simulink model "gm_parallel_lht"  (R2019b)
settings: Solver=FixedStepDiscrete  StartTime=0.0  StopTime=inf  RelTol=1e-3
undefined symbols (not defined in the file or in its folder): bt, height, width
libraries: hdlsllib x190, simulink x13, hdlmdlgenlib x7, dspsrcs4 x1
(part 15 of 18)

== system gm_parallel_lht/Parallel LHT/Parallel LHT Accumulator/Accumulator with Switches/Accumulator_instance35/Block RAM/Simple Dual Port RAM ==
  wr_data : Inport  OutDataTypeStr=fixdt(0, 11, 0)  PortDimensions=1  SampleTime=6.66666666666667e-09
  wr_addr : Inport  Port=2  OutDataTypeStr=fixdt(0, 11, 0)  PortDimensions=1  SampleTime=6.66666666666667e-09
  wr_en : Inport  Port=3  OutDataTypeStr=boolean  PortDimensions=1  SampleTime=6.66666666666667e-09
  rd_addr : Inport  Port=4  OutDataTypeStr=fixdt(0, 11, 0)  PortDimensions=1  SampleTime=6.66666666666667e-09
  Simple Dual Port RAM : hdlsllib/HDL RAMs/Simple Dual Port RAM  ram_size=ceil(log2(maxRho*2))
      settings: SourceProductName=Simulink  SourceProductBaseCode=SL
  rd_data : Outport
  wires:
  rd_addr/1 -> Simple Dual Port RAM/4
  wr_en/1 -> Simple Dual Port RAM/3
  wr_addr/1 -> Simple Dual Port RAM/2
  wr_data/1 -> Simple Dual Port RAM/1
  Simple Dual Port RAM/1 -> rd_data/1

== system gm_parallel_lht/Parallel LHT/Parallel LHT Accumulator/Accumulator with Switches/Accumulator_instance36/Block RAM/Simple Dual Port RAM ==
  wr_data : Inport  OutDataTypeStr=fixdt(0, 11, 0)  PortDimensions=1  SampleTime=6.66666666666667e-09
  wr_addr : Inport  Port=2  OutDataTypeStr=fixdt(0, 11, 0)  PortDimensions=1  SampleTime=6.66666666666667e-09
  wr_en : Inport  Port=3  OutDataTypeStr=boolean  PortDimensions=1  SampleTime=6.66666666666667e-09
  rd_addr : Inport  Port=4  OutDataTypeStr=fixdt(0, 11, 0)  PortDimensions=1  SampleTime=6.66666666666667e-09
  Simple Dual Port RAM : hdlsllib/HDL RAMs/Simple Dual Port RAM  ram_size=ceil(log2(maxRho*2))
      settings: SourceProductName=Simulink  SourceProductBaseCode=SL
  rd_data : Outport
  wires:
  rd_addr/1 -> Simple Dual Port RAM/4
  wr_en/1 -> Simple Dual Port RAM/3
  wr_addr/1 -> Simple Dual Port RAM/2
  wr_data/1 -> Simple Dual Port RAM/1
  Simple Dual Port RAM/1 -> rd_data/1

== system gm_parallel_lht/Parallel LHT/Parallel LHT Accumulator/Accumulator with Switches/Accumulator_instance37/Block RAM/Simple Dual Port RAM ==
  wr_data : Inport  OutDataTypeStr=fixdt(0, 11, 0)  PortDimensions=1  SampleTime=6.66666666666667e-09
  wr_addr : Inport  Port=2  OutDataTypeStr=fixdt(0, 11, 0)  PortDimensions=1  SampleTime=6.66666666666667e-09
  wr_en : Inport  Port=3  OutDataTypeStr=boolean  PortDimensions=1  SampleTime=6.66666666666667e-09
  rd_addr : Inport  Port=4  OutDataTypeStr=fixdt(0, 11, 0)  PortDimensions=1  SampleTime=6.66666666666667e-09
  Simple Dual Port RAM : hdlsllib/HDL RAMs/Simple Dual Port RAM  ram_size=ceil(log2(maxRho*2))
      settings: SourceProductName=Simulink  SourceProductBaseCode=SL
  rd_data : Outport
  wires:
  rd_addr/1 -> Simple Dual Port RAM/4
  wr_en/1 -> Simple Dual Port RAM/3
  wr_addr/1 -> Simple Dual Port RAM/2
  wr_data/1 -> Simple Dual Port RAM/1
  Simple Dual Port RAM/1 -> rd_data/1

== system gm_parallel_lht/Parallel LHT/Parallel LHT Accumulator/Accumulator with Switches/Accumulator_instance38/Block RAM/Simple Dual Port RAM ==
  wr_data : Inport  OutDataTypeStr=fixdt(0, 11, 0)  PortDimensions=1  SampleTime=6.66666666666667e-09
  wr_addr : Inport  Port=2  OutDataTypeStr=fixdt(0, 11, 0)  PortDimensions=1  SampleTime=6.66666666666667e-09
  wr_en : Inport  Port=3  OutDataTypeStr=boolean  PortDimensions=1  SampleTime=6.66666666666667e-09
  rd_addr : Inport  Port=4  OutDataTypeStr=fixdt(0, 11, 0)  PortDimensions=1  SampleTime=6.66666666666667e-09
  Simple Dual Port RAM : hdlsllib/HDL RAMs/Simple Dual Port RAM  ram_size=ceil(log2(maxRho*2))
      settings: SourceProductName=Simulink  SourceProductBaseCode=SL
  rd_data : Outport
  wires:
  rd_addr/1 -> Simple Dual Port RAM/4
  wr_en/1 -> Simple Dual Port RAM/3
  wr_addr/1 -> Simple Dual Port RAM/2
  wr_data/1 -> Simple Dual Port RAM/1
  Simple Dual Port RAM/1 -> rd_data/1

== system gm_parallel_lht/Parallel LHT/Parallel LHT Accumulator/Accumulator with Switches/Accumulator_instance39/Block RAM/Simple Dual Port RAM ==
  wr_data : Inport  OutDataTypeStr=fixdt(0, 11, 0)  PortDimensions=1  SampleTime=6.66666666666667e-09
  wr_addr : Inport  Port=2  OutDataTypeStr=fixdt(0, 11, 0)  PortDimensions=1  SampleTime=6.66666666666667e-09
  wr_en : Inport  Port=3  OutDataTypeStr=boolean  PortDimensions=1  SampleTime=6.66666666666667e-09
  rd_addr : Inport  Port=4  OutDataTypeStr=fixdt(0, 11, 0)  PortDimensions=1  SampleTime=6.66666666666667e-09
  Simple Dual Port RAM : hdlsllib/HDL RAMs/Simple Dual Port RAM  ram_size=ceil(log2(maxRho*2))
      settings: SourceProductName=Simulink  SourceProductBaseCode=SL
  rd_data : Outport
  wires:
  rd_addr/1 -> Simple Dual Port RAM/4
  wr_en/1 -> Simple Dual Port RAM/3
  wr_addr/1 -> Simple Dual Port RAM/2
  wr_data/1 -> Simple Dual Port RAM/1
  Simple Dual Port RAM/1 -> rd_data/1

== system gm_parallel_lht/Parallel LHT/Parallel LHT Accumulator/Accumulator with Switches/Accumulator_instance4/Block RAM/Simple Dual Port RAM ==
  wr_data : Inport  OutDataTypeStr=fixdt(0, 11, 0)  PortDimensions=1  SampleTime=6.66666666666667e-09
  wr_addr : Inport  Port=2  OutDataTypeStr=fixdt(0, 11, 0)  PortDimensions=1  SampleTime=6.66666666666667e-09
  wr_en : Inport  Port=3  OutDataTypeStr=boolean  PortDimensions=1  SampleTime=6.66666666666667e-09
  rd_addr : Inport  Port=4  OutDataTypeStr=fixdt(0, 11, 0)  PortDimensions=1  SampleTime=6.66666666666667e-09
  Simple Dual Port RAM : hdlsllib/HDL RAMs/Simple Dual Port RAM  ram_size=ceil(log2(maxRho*2))
      settings: SourceProductName=Simulink  SourceProductBaseCode=SL
  rd_data : Outport
  wires:
  rd_addr/1 -> Simple Dual Port RAM/4
  wr_en/1 -> Simple Dual Port RAM/3
  wr_addr/1 -> Simple Dual Port RAM/2
  wr_data/1 -> Simple Dual Port RAM/1
  Simple Dual Port RAM/1 -> rd_data/1

== system gm_parallel_lht/Parallel LHT/Parallel LHT Accumulator/Accumulator with Switches/Accumulator_instance40/Block RAM/Simple Dual Port RAM ==
  wr_data : Inport  OutDataTypeStr=fixdt(0, 11, 0)  PortDimensions=1  SampleTime=6.66666666666667e-09
  wr_addr : Inport  Port=2  OutDataTypeStr=fixdt(0, 11, 0)  PortDimensions=1  SampleTime=6.66666666666667e-09
  wr_en : Inport  Port=3  OutDataTypeStr=boolean  PortDimensions=1  SampleTime=6.66666666666667e-09
  rd_addr : Inport  Port=4  OutDataTypeStr=fixdt(0, 11, 0)  PortDimensions=1  SampleTime=6.66666666666667e-09
  Simple Dual Port RAM : hdlsllib/HDL RAMs/Simple Dual Port RAM  ram_size=ceil(log2(maxRho*2))
      settings: SourceProductName=Simulink  SourceProductBaseCode=SL
  rd_data : Outport
  wires:
  rd_addr/1 -> Simple Dual Port RAM/4
  wr_en/1 -> Simple Dual Port RAM/3
  wr_addr/1 -> Simple Dual Port RAM/2
  wr_data/1 -> Simple Dual Port RAM/1
  Simple Dual Port RAM/1 -> rd_data/1

== system gm_parallel_lht/Parallel LHT/Parallel LHT Accumulator/Accumulator with Switches/Accumulator_instance41/Block RAM/Simple Dual Port RAM ==
  wr_data : Inport  OutDataTypeStr=fixdt(0, 11, 0)  PortDimensions=1  SampleTime=6.66666666666667e-09
  wr_addr : Inport  Port=2  OutDataTypeStr=fixdt(0, 11, 0)  PortDimensions=1  SampleTime=6.66666666666667e-09
  wr_en : Inport  Port=3  OutDataTypeStr=boolean  PortDimensions=1  SampleTime=6.66666666666667e-09
  rd_addr : Inport  Port=4  OutDataTypeStr=fixdt(0, 11, 0)  PortDimensions=1  SampleTime=6.66666666666667e-09
  Simple Dual Port RAM : hdlsllib/HDL RAMs/Simple Dual Port RAM  ram_size=ceil(log2(maxRho*2))
      settings: SourceProductName=Simulink  SourceProductBaseCode=SL
  rd_data : Outport
  wires:
  rd_addr/1 -> Simple Dual Port RAM/4
  wr_en/1 -> Simple Dual Port RAM/3
  wr_addr/1 -> Simple Dual Port RAM/2
  wr_data/1 -> Simple Dual Port RAM/1
  Simple Dual Port RAM/1 -> rd_data/1

== system gm_parallel_lht/Parallel LHT/Parallel LHT Accumulator/Accumulator with Switches/Accumulator_instance42/Block RAM/Simple Dual Port RAM ==
  wr_data : Inport  OutDataTypeStr=fixdt(0, 11, 0)  PortDimensions=1  SampleTime=6.66666666666667e-09
  wr_addr : Inport  Port=2  OutDataTypeStr=fixdt(0, 11, 0)  PortDimensions=1  SampleTime=6.66666666666667e-09
  wr_en : Inport  Port=3  OutDataTypeStr=boolean  PortDimensions=1  SampleTime=6.66666666666667e-09
  rd_addr : Inport  Port=4  OutDataTypeStr=fixdt(0, 11, 0)  PortDimensions=1  SampleTime=6.66666666666667e-09
  Simple Dual Port RAM : hdlsllib/HDL RAMs/Simple Dual Port RAM  ram_size=ceil(log2(maxRho*2))
      settings: SourceProductName=Simulink  SourceProductBaseCode=SL
  rd_data : Outport
  wires:
  rd_addr/1 -> Simple Dual Port RAM/4
  wr_en/1 -> Simple Dual Port RAM/3
  wr_addr/1 -> Simple Dual Port RAM/2
  wr_data/1 -> Simple Dual Port RAM/1
  Simple Dual Port RAM/1 -> rd_data/1

== system gm_parallel_lht/Parallel LHT/Parallel LHT Accumulator/Accumulator with Switches/Accumulator_instance43/Block RAM/Simple Dual Port RAM ==
  wr_data : Inport  OutDataTypeStr=fixdt(0, 11, 0)  PortDimensions=1  SampleTime=6.66666666666667e-09
  wr_addr : Inport  Port=2  OutDataTypeStr=fixdt(0, 11, 0)  PortDimensions=1  SampleTime=6.66666666666667e-09
  wr_en : Inport  Port=3  OutDataTypeStr=boolean  PortDimensions=1  SampleTime=6.66666666666667e-09
  rd_addr : Inport  Port=4  OutDataTypeStr=fixdt(0, 11, 0)  PortDimensions=1  SampleTime=6.66666666666667e-09
  Simple Dual Port RAM : hdlsllib/HDL RAMs/Simple Dual Port RAM  ram_size=ceil(log2(maxRho*2))
      settings: SourceProductName=Simulink  SourceProductBaseCode=SL
  rd_data : Outport
  wires:
  rd_addr/1 -> Simple Dual Port RAM/4
  wr_en/1 -> Simple Dual Port RAM/3
  wr_addr/1 -> Simple Dual Port RAM/2
  wr_data/1 -> Simple Dual Port RAM/1
  Simple Dual Port RAM/1 -> rd_data/1

== system gm_parallel_lht/Parallel LHT/Parallel LHT Accumulator/Accumulator with Switches/Accumulator_instance44/Block RAM/Simple Dual Port RAM ==
  wr_data : Inport  OutDataTypeStr=fixdt(0, 11, 0)  PortDimensions=1  SampleTime=6.66666666666667e-09
  wr_addr : Inport  Port=2  OutDataTypeStr=fixdt(0, 11, 0)  PortDimensions=1  SampleTime=6.66666666666667e-09
  wr_en : Inport  Port=3  OutDataTypeStr=boolean  PortDimensions=1  SampleTime=6.66666666666667e-09
  rd_addr : Inport  Port=4  OutDataTypeStr=fixdt(0, 11, 0)  PortDimensions=1  SampleTime=6.66666666666667e-09
  Simple Dual Port RAM : hdlsllib/HDL RAMs/Simple Dual Port RAM  ram_size=ceil(log2(maxRho*2))
      settings: SourceProductName=Simulink  SourceProductBaseCode=SL
  rd_data : Outport
  wires:
  rd_addr/1 -> Simple Dual Port RAM/4
  wr_en/1 -> Simple Dual Port RAM/3
  wr_addr/1 -> Simple Dual Port RAM/2
  wr_data/1 -> Simple Dual Port RAM/1
  Simple Dual Port RAM/1 -> rd_data/1

== system gm_parallel_lht/Parallel LHT/Parallel LHT Accumulator/Accumulator with Switches/Accumulator_instance45/Block RAM/Simple Dual Port RAM ==
  wr_data : Inport  OutDataTypeStr=fixdt(0, 11, 0)  PortDimensions=1  SampleTime=6.66666666666667e-09
  wr_addr : Inport  Port=2  OutDataTypeStr=fixdt(0, 11, 0)  PortDimensions=1  SampleTime=6.66666666666667e-09
  wr_en : Inport  Port=3  OutDataTypeStr=boolean  PortDimensions=1  SampleTime=6.66666666666667e-09
  rd_addr : Inport  Port=4  OutDataTypeStr=fixdt(0, 11, 0)  PortDimensions=1  SampleTime=6.66666666666667e-09
  Simple Dual Port RAM : hdlsllib/HDL RAMs/Simple Dual Port RAM  ram_size=ceil(log2(maxRho*2))
      settings: SourceProductName=Simulink  SourceProductBaseCode=SL
  rd_data : Outport
  wires:
  rd_addr/1 -> Simple Dual Port RAM/4
  wr_en/1 -> Simple Dual Port RAM/3
  wr_addr/1 -> Simple Dual Port RAM/2
  wr_data/1 -> Simple Dual Port RAM/1
  Simple Dual Port RAM/1 -> rd_data/1

== system gm_parallel_lht/Parallel LHT/Parallel LHT Accumulator/Accumulator with Switches/Accumulator_instance46/Block RAM/Simple Dual Port RAM ==
  wr_data : Inport  OutDataTypeStr=fixdt(0, 11, 0)  PortDimensions=1  SampleTime=6.66666666666667e-09
  wr_addr : Inport  Port=2  OutDataTypeStr=fixdt(0, 11, 0)  PortDimensions=1  SampleTime=6.66666666666667e-09
  wr_en : Inport  Port=3  OutDataTypeStr=boolean  PortDimensions=1  SampleTime=6.66666666666667e-09
  rd_addr : Inport  Port=4  OutDataTypeStr=fixdt(0, 11, 0)  PortDimensions=1  SampleTime=6.66666666666667e-09
  Simple Dual Port RAM : hdlsllib/HDL RAMs/Simple Dual Port RAM  ram_size=ceil(log2(maxRho*2))
      settings: SourceProductName=Simulink  SourceProductBaseCode=SL
  rd_data : Outport
  wires:
  rd_addr/1 -> Simple Dual Port RAM/4
  wr_en/1 -> Simple Dual Port RAM/3
  wr_addr/1 -> Simple Dual Port RAM/2
  wr_data/1 -> Simple Dual Port RAM/1
  Simple Dual Port RAM/1 -> rd_data/1

== system gm_parallel_lht/Parallel LHT/Parallel LHT Accumulator/Accumulator with Switches/Accumulator_instance47/Block RAM/Simple Dual Port RAM ==
  wr_data : Inport  OutDataTypeStr=fixdt(0, 11, 0)  PortDimensions=1  SampleTime=6.66666666666667e-09
  wr_addr : Inport  Port=2  OutDataTypeStr=fixdt(0, 11, 0)  PortDimensions=1  SampleTime=6.66666666666667e-09
  wr_en : Inport  Port=3  OutDataTypeStr=boolean  PortDimensions=1  SampleTime=6.66666666666667e-09
  rd_addr : Inport  Port=4  OutDataTypeStr=fixdt(0, 11, 0)  PortDimensions=1  SampleTime=6.66666666666667e-09
  Simple Dual Port RAM : hdlsllib/HDL RAMs/Simple Dual Port RAM  ram_size=ceil(log2(maxRho*2))
      settings: SourceProductName=Simulink  SourceProductBaseCode=SL
  rd_data : Outport
  wires:
  rd_addr/1 -> Simple Dual Port RAM/4
  wr_en/1 -> Simple Dual Port RAM/3
  wr_addr/1 -> Simple Dual Port RAM/2
  wr_data/1 -> Simple Dual Port RAM/1
  Simple Dual Port RAM/1 -> rd_data/1

== system gm_parallel_lht/Parallel LHT/Parallel LHT Accumulator/Accumulator with Switches/Accumulator_instance48/Block RAM/Simple Dual Port RAM ==
  wr_data : Inport  OutDataTypeStr=fixdt(0, 11, 0)  PortDimensions=1  SampleTime=6.66666666666667e-09
  wr_addr : Inport  Port=2  OutDataTypeStr=fixdt(0, 11, 0)  PortDimensions=1  SampleTime=6.66666666666667e-09
  wr_en : Inport  Port=3  OutDataTypeStr=boolean  PortDimensions=1  SampleTime=6.66666666666667e-09
  rd_addr : Inport  Port=4  OutDataTypeStr=fixdt(0, 11, 0)  PortDimensions=1  SampleTime=6.66666666666667e-09
  Simple Dual Port RAM : hdlsllib/HDL RAMs/Simple Dual Port RAM  ram_size=ceil(log2(maxRho*2))
      settings: SourceProductName=Simulink  SourceProductBaseCode=SL
  rd_data : Outport
  wires:
  rd_addr/1 -> Simple Dual Port RAM/4
  wr_en/1 -> Simple Dual Port RAM/3
  wr_addr/1 -> Simple Dual Port RAM/2
  wr_data/1 -> Simple Dual Port RAM/1
  Simple Dual Port RAM/1 -> rd_data/1

== system gm_parallel_lht/Parallel LHT/Parallel LHT Accumulator/Accumulator with Switches/Accumulator_instance49/Block RAM/Simple Dual Port RAM ==
  wr_data : Inport  OutDataTypeStr=fixdt(0, 11, 0)  PortDimensions=1  SampleTime=6.66666666666667e-09
  wr_addr : Inport  Port=2  OutDataTypeStr=fixdt(0, 11, 0)  PortDimensions=1  SampleTime=6.66666666666667e-09
  wr_en : Inport  Port=3  OutDataTypeStr=boolean  PortDimensions=1  SampleTime=6.66666666666667e-09
  rd_addr : Inport  Port=4  OutDataTypeStr=fixdt(0, 11, 0)  PortDimensions=1  SampleTime=6.66666666666667e-09
  Simple Dual Port RAM : hdlsllib/HDL RAMs/Simple Dual Port RAM  ram_size=ceil(log2(maxRho*2))
      settings: SourceProductName=Simulink  SourceProductBaseCode=SL
  rd_data : Outport
  wires:
  rd_addr/1 -> Simple Dual Port RAM/4
  wr_en/1 -> Simple Dual Port RAM/3
  wr_addr/1 -> Simple Dual Port RAM/2
  wr_data/1 -> Simple Dual Port RAM/1
  Simple Dual Port RAM/1 -> rd_data/1

== system gm_parallel_lht/Parallel LHT/Parallel LHT Accumulator/Accumulator with Switches/Accumulator_instance5/Block RAM/Simple Dual Port RAM ==
  wr_data : Inport  OutDataTypeStr=fixdt(0, 11, 0)  PortDimensions=1  SampleTime=6.66666666666667e-09
  wr_addr : Inport  Port=2  OutDataTypeStr=fixdt(0, 11, 0)  PortDimensions=1  SampleTime=6.66666666666667e-09
  wr_en : Inport  Port=3  OutDataTypeStr=boolean  PortDimensions=1  SampleTime=6.66666666666667e-09
  rd_addr : Inport  Port=4  OutDataTypeStr=fixdt(0, 11, 0)  PortDimensions=1  SampleTime=6.66666666666667e-09
  Simple Dual Port RAM : hdlsllib/HDL RAMs/Simple Dual Port RAM  ram_size=ceil(log2(maxRho*2))
      settings: SourceProductName=Simulink  SourceProductBaseCode=SL
  rd_data : Outport
  wires:
  rd_addr/1 -> Simple Dual Port RAM/4
  wr_en/1 -> Simple Dual Port RAM/3
  wr_addr/1 -> Simple Dual Port RAM/2
  wr_data/1 -> Simple Dual Port RAM/1
  Simple Dual Port RAM/1 -> rd_data/1

== system gm_parallel_lht/Parallel LHT/Parallel LHT Accumulator/Accumulator with Switches/Accumulator_instance50/Block RAM/Simple Dual Port RAM ==
  wr_data : Inport  OutDataTypeStr=fixdt(0, 11, 0)  PortDimensions=1  SampleTime=6.66666666666667e-09
  wr_addr : Inport  Port=2  OutDataTypeStr=fixdt(0, 11, 0)  PortDimensions=1  SampleTime=6.66666666666667e-09
  wr_en : Inport  Port=3  OutDataTypeStr=boolean  PortDimensions=1  SampleTime=6.66666666666667e-09
  rd_addr : Inport  Port=4  OutDataTypeStr=fixdt(0, 11, 0)  PortDimensions=1  SampleTime=6.66666666666667e-09
  Simple Dual Port RAM : hdlsllib/HDL RAMs/Simple Dual Port RAM  ram_size=ceil(log2(maxRho*2))
      settings: SourceProductName=Simulink  SourceProductBaseCode=SL
  rd_data : Outport
  wires:
  rd_addr/1 -> Simple Dual Port RAM/4
  wr_en/1 -> Simple Dual Port RAM/3
  wr_addr/1 -> Simple Dual Port RAM/2
  wr_data/1 -> Simple Dual Port RAM/1
  Simple Dual Port RAM/1 -> rd_data/1

== system gm_parallel_lht/Parallel LHT/Parallel LHT Accumulator/Accumulator with Switches/Accumulator_instance51/Block RAM/Simple Dual Port RAM ==
  wr_data : Inport  OutDataTypeStr=fixdt(0, 11, 0)  PortDimensions=1  SampleTime=6.66666666666667e-09
  wr_addr : Inport  Port=2  OutDataTypeStr=fixdt(0, 11, 0)  PortDimensions=1  SampleTime=6.66666666666667e-09
  wr_en : Inport  Port=3  OutDataTypeStr=boolean  PortDimensions=1  SampleTime=6.66666666666667e-09
  rd_addr : Inport  Port=4  OutDataTypeStr=fixdt(0, 11, 0)  PortDimensions=1  SampleTime=6.66666666666667e-09
  Simple Dual Port RAM : hdlsllib/HDL RAMs/Simple Dual Port RAM  ram_size=ceil(log2(maxRho*2))
      settings: SourceProductName=Simulink  SourceProductBaseCode=SL
  rd_data : Outport
  wires:
  rd_addr/1 -> Simple Dual Port RAM/4
  wr_en/1 -> Simple Dual Port RAM/3
  wr_addr/1 -> Simple Dual Port RAM/2
  wr_data/1 -> Simple Dual Port RAM/1
  Simple Dual Port RAM/1 -> rd_data/1

== system gm_parallel_lht/Parallel LHT/Parallel LHT Accumulator/Accumulator with Switches/Accumulator_instance52/Block RAM/Simple Dual Port RAM ==
  wr_data : Inport  OutDataTypeStr=fixdt(0, 11, 0)  PortDimensions=1  SampleTime=6.66666666666667e-09
  wr_addr : Inport  Port=2  OutDataTypeStr=fixdt(0, 11, 0)  PortDimensions=1  SampleTime=6.66666666666667e-09
  wr_en : Inport  Port=3  OutDataTypeStr=boolean  PortDimensions=1  SampleTime=6.66666666666667e-09
  rd_addr : Inport  Port=4  OutDataTypeStr=fixdt(0, 11, 0)  PortDimensions=1  SampleTime=6.66666666666667e-09
  Simple Dual Port RAM : hdlsllib/HDL RAMs/Simple Dual Port RAM  ram_size=ceil(log2(maxRho*2))
      settings: SourceProductName=Simulink  SourceProductBaseCode=SL
  rd_data : Outport
  wires:
  rd_addr/1 -> Simple Dual Port RAM/4
  wr_en/1 -> Simple Dual Port RAM/3
  wr_addr/1 -> Simple Dual Port RAM/2
  wr_data/1 -> Simple Dual Port RAM/1
  Simple Dual Port RAM/1 -> rd_data/1

== system gm_parallel_lht/Parallel LHT/Parallel LHT Accumulator/Accumulator with Switches/Accumulator_instance53/Block RAM/Simple Dual Port RAM ==
  wr_data : Inport  OutDataTypeStr=fixdt(0, 11, 0)  PortDimensions=1  SampleTime=6.66666666666667e-09
  wr_addr : Inport  Port=2  OutDataTypeStr=fixdt(0, 11, 0)  PortDimensions=1  SampleTime=6.66666666666667e-09
  wr_en : Inport  Port=3  OutDataTypeStr=boolean  PortDimensions=1  SampleTime=6.66666666666667e-09
  rd_addr : Inport  Port=4  OutDataTypeStr=fixdt(0, 11, 0)  PortDimensions=1  SampleTime=6.66666666666667e-09
  Simple Dual Port RAM : hdlsllib/HDL RAMs/Simple Dual Port RAM  ram_size=ceil(log2(maxRho*2))
      settings: SourceProductName=Simulink  SourceProductBaseCode=SL
  rd_data : Outport
  wires:
  rd_addr/1 -> Simple Dual Port RAM/4
  wr_en/1 -> Simple Dual Port RAM/3
  wr_addr/1 -> Simple Dual Port RAM/2
  wr_data/1 -> Simple Dual Port RAM/1
  Simple Dual Port RAM/1 -> rd_data/1

== system gm_parallel_lht/Parallel LHT/Parallel LHT Accumulator/Accumulator with Switches/Accumulator_instance54/Block RAM/Simple Dual Port RAM ==
  wr_data : Inport  OutDataTypeStr=fixdt(0, 11, 0)  PortDimensions=1  SampleTime=6.66666666666667e-09
  wr_addr : Inport  Port=2  OutDataTypeStr=fixdt(0, 11, 0)  PortDimensions=1  SampleTime=6.66666666666667e-09
  wr_en : Inport  Port=3  OutDataTypeStr=boolean  PortDimensions=1  SampleTime=6.66666666666667e-09
  rd_addr : Inport  Port=4  OutDataTypeStr=fixdt(0, 11, 0)  PortDimensions=1  SampleTime=6.66666666666667e-09
  Simple Dual Port RAM : hdlsllib/HDL RAMs/Simple Dual Port RAM  ram_size=ceil(log2(maxRho*2))
      settings: SourceProductName=Simulink  SourceProductBaseCode=SL
  rd_data : Outport
  wires:
  rd_addr/1 -> Simple Dual Port RAM/4
  wr_en/1 -> Simple Dual Port RAM/3
  wr_addr/1 -> Simple Dual Port RAM/2
  wr_data/1 -> Simple Dual Port RAM/1
  Simple Dual Port RAM/1 -> rd_data/1

== system gm_parallel_lht/Parallel LHT/Parallel LHT Accumulator/Accumulator with Switches/Accumulator_instance55/Block RAM/Simple Dual Port RAM ==
  wr_data : Inport  OutDataTypeStr=fixdt(0, 11, 0)  PortDimensions=1  SampleTime=6.66666666666667e-09
  wr_addr : Inport  Port=2  OutDataTypeStr=fixdt(0, 11, 0)  PortDimensions=1  SampleTime=6.66666666666667e-09
  wr_en : Inport  Port=3  OutDataTypeStr=boolean  PortDimensions=1  SampleTime=6.66666666666667e-09
  rd_addr : Inport  Port=4  OutDataTypeStr=fixdt(0, 11, 0)  PortDimensions=1  SampleTime=6.66666666666667e-09
  Simple Dual Port RAM : hdlsllib/HDL RAMs/Simple Dual Port RAM  ram_size=ceil(log2(maxRho*2))
      settings: SourceProductName=Simulink  SourceProductBaseCode=SL
  rd_data : Outport
  wires:
  rd_addr/1 -> Simple Dual Port RAM/4
  wr_en/1 -> Simple Dual Port RAM/3
  wr_addr/1 -> Simple Dual Port RAM/2
  wr_data/1 -> Simple Dual Port RAM/1
  Simple Dual Port RAM/1 -> rd_data/1

== system gm_parallel_lht/Parallel LHT/Parallel LHT Accumulator/Accumulator with Switches/Accumulator_instance56/Block RAM/Simple Dual Port RAM ==
  wr_data : Inport  OutDataTypeStr=fixdt(0, 11, 0)  PortDimensions=1  SampleTime=6.66666666666667e-09
  wr_addr : Inport  Port=2  OutDataTypeStr=fixdt(0, 11, 0)  PortDimensions=1  SampleTime=6.66666666666667e-09
  wr_en : Inport  Port=3  OutDataTypeStr=boolean  PortDimensions=1  SampleTime=6.66666666666667e-09
  rd_addr : Inport  Port=4  OutDataTypeStr=fixdt(0, 11, 0)  PortDimensions=1  SampleTime=6.66666666666667e-09
  Simple Dual Port RAM : hdlsllib/HDL RAMs/Simple Dual Port RAM  ram_size=ceil(log2(maxRho*2))
      settings: SourceProductName=Simulink  SourceProductBaseCode=SL
  rd_data : Outport
  wires:
  rd_addr/1 -> Simple Dual Port RAM/4
  wr_en/1 -> Simple Dual Port RAM/3
  wr_addr/1 -> Simple Dual Port RAM/2
  wr_data/1 -> Simple Dual Port RAM/1
  Simple Dual Port RAM/1 -> rd_data/1

== system gm_parallel_lht/Parallel LHT/Parallel LHT Accumulator/Accumulator with Switches/Accumulator_instance57/Block RAM/Simple Dual Port RAM ==
  wr_data : Inport  OutDataTypeStr=fixdt(0, 11, 0)  PortDimensions=1  SampleTime=6.66666666666667e-09
  wr_addr : Inport  Port=2  OutDataTypeStr=fixdt(0, 11, 0)  PortDimensions=1  SampleTime=6.66666666666667e-09
  wr_en : Inport  Port=3  OutDataTypeStr=boolean  PortDimensions=1  SampleTime=6.66666666666667e-09
  rd_addr : Inport  Port=4  OutDataTypeStr=fixdt(0, 11, 0)  PortDimensions=1  SampleTime=6.66666666666667e-09
  Simple Dual Port RAM : hdlsllib/HDL RAMs/Simple Dual Port RAM  ram_size=ceil(log2(maxRho*2))
      settings: SourceProductName=Simulink  SourceProductBaseCode=SL
  rd_data : Outport
  wires:
  rd_addr/1 -> Simple Dual Port RAM/4
  wr_en/1 -> Simple Dual Port RAM/3
  wr_addr/1 -> Simple Dual Port RAM/2
  wr_data/1 -> Simple Dual Port RAM/1
  Simple Dual Port RAM/1 -> rd_data/1

== system gm_parallel_lht/Parallel LHT/Parallel LHT Accumulator/Accumulator with Switches/Accumulator_instance58/Block RAM/Simple Dual Port RAM ==
  wr_data : Inport  OutDataTypeStr=fixdt(0, 11, 0)  PortDimensions=1  SampleTime=6.66666666666667e-09
  wr_addr : Inport  Port=2  OutDataTypeStr=fixdt(0, 11, 0)  PortDimensions=1  SampleTime=6.66666666666667e-09
  wr_en : Inport  Port=3  OutDataTypeStr=boolean  PortDimensions=1  SampleTime=6.66666666666667e-09
  rd_addr : Inport  Port=4  OutDataTypeStr=fixdt(0, 11, 0)  PortDimensions=1  SampleTime=6.66666666666667e-09
  Simple Dual Port RAM : hdlsllib/HDL RAMs/Simple Dual Port RAM  ram_size=ceil(log2(maxRho*2))
      settings: SourceProductName=Simulink  SourceProductBaseCode=SL
  rd_data : Outport
  wires:
  rd_addr/1 -> Simple Dual Port RAM/4
  wr_en/1 -> Simple Dual Port RAM/3
  wr_addr/1 -> Simple Dual Port RAM/2
  wr_data/1 -> Simple Dual Port RAM/1
  Simple Dual Port RAM/1 -> rd_data/1

== system gm_parallel_lht/Parallel LHT/Parallel LHT Accumulator/Accumulator with Switches/Accumulator_instance59/Block RAM/Simple Dual Port RAM ==
  wr_data : Inport  OutDataTypeStr=fixdt(0, 11, 0)  PortDimensions=1  SampleTime=6.66666666666667e-09
  wr_addr : Inport  Port=2  OutDataTypeStr=fixdt(0, 11, 0)  PortDimensions=1  SampleTime=6.66666666666667e-09
  wr_en : Inport  Port=3  OutDataTypeStr=boolean  PortDimensions=1  SampleTime=6.66666666666667e-09
  rd_addr : Inport  Port=4  OutDataTypeStr=fixdt(0, 11, 0)  PortDimensions=1  SampleTime=6.66666666666667e-09
  Simple Dual Port RAM : hdlsllib/HDL RAMs/Simple Dual Port RAM  ram_size=ceil(log2(maxRho*2))
      settings: SourceProductName=Simulink  SourceProductBaseCode=SL
  rd_data : Outport
  wires:
  rd_addr/1 -> Simple Dual Port RAM/4
  wr_en/1 -> Simple Dual Port RAM/3
  wr_addr/1 -> Simple Dual Port RAM/2
  wr_data/1 -> Simple Dual Port RAM/1
  Simple Dual Port RAM/1 -> rd_data/1

== system gm_parallel_lht/Parallel LHT/Parallel LHT Accumulator/Accumulator with Switches/Accumulator_instance6/Block RAM/Simple Dual Port RAM ==
  wr_data : Inport  OutDataTypeStr=fixdt(0, 11, 0)  PortDimensions=1  SampleTime=6.66666666666667e-09
  wr_addr : Inport  Port=2  OutDataTypeStr=fixdt(0, 11, 0)  PortDimensions=1  SampleTime=6.66666666666667e-09
  wr_en : Inport  Port=3  OutDataTypeStr=boolean  PortDimensions=1  SampleTime=6.66666666666667e-09
  rd_addr : Inport  Port=4  OutDataTypeStr=fixdt(0, 11, 0)  PortDimensions=1  SampleTime=6.66666666666667e-09
  Simple Dual Port RAM : hdlsllib/HDL RAMs/Simple Dual Port RAM  ram_size=ceil(log2(maxRho*2))
      settings: SourceProductName=Simulink  SourceProductBaseCode=SL
  rd_data : Outport
  wires:
  rd_addr/1 -> Simple Dual Port RAM/4
  wr_en/1 -> Simple Dual Port RAM/3
  wr_addr/1 -> Simple Dual Port RAM/2
  wr_data/1 -> Simple Dual Port RAM/1
  Simple Dual Port RAM/1 -> rd_data/1

== system gm_parallel_lht/Parallel LHT/Parallel LHT Accumulator/Accumulator with Switches/Accumulator_instance60/Block RAM/Simple Dual Port RAM ==
  wr_data : Inport  OutDataTypeStr=fixdt(0, 11, 0)  PortDimensions=1  SampleTime=6.66666666666667e-09
  wr_addr : Inport  Port=2  OutDataTypeStr=fixdt(0, 11, 0)  PortDimensions=1  SampleTime=6.66666666666667e-09
  wr_en : Inport  Port=3  OutDataTypeStr=boolean  PortDimensions=1  SampleTime=6.66666666666667e-09
  rd_addr : Inport  Port=4  OutDataTypeStr=fixdt(0, 11, 0)  PortDimensions=1  SampleTime=6.66666666666667e-09
  Simple Dual Port RAM : hdlsllib/HDL RAMs/Simple Dual Port RAM  ram_size=ceil(log2(maxRho*2))
      settings: SourceProductName=Simulink  SourceProductBaseCode=SL
  rd_data : Outport
  wires:
  rd_addr/1 -> Simple Dual Port RAM/4
  wr_en/1 -> Simple Dual Port RAM/3
  wr_addr/1 -> Simple Dual Port RAM/2
  wr_data/1 -> Simple Dual Port RAM/1
  Simple Dual Port RAM/1 -> rd_data/1

== system gm_parallel_lht/Parallel LHT/Parallel LHT Accumulator/Accumulator with Switches/Accumulator_instance61/Block RAM/Simple Dual Port RAM ==
  wr_data : Inport  OutDataTypeStr=fixdt(0, 11, 0)  PortDimensions=1  SampleTime=6.66666666666667e-09
  wr_addr : Inport  Port=2  OutDataTypeStr=fixdt(0, 11, 0)  PortDimensions=1  SampleTime=6.66666666666667e-09
  wr_en : Inport  Port=3  OutDataTypeStr=boolean  PortDimensions=1  SampleTime=6.66666666666667e-09
  rd_addr : Inport  Port=4  OutDataTypeStr=fixdt(0, 11, 0)  PortDimensions=1  SampleTime=6.66666666666667e-09
  Simple Dual Port RAM : hdlsllib/HDL RAMs/Simple Dual Port RAM  ram_size=ceil(log2(maxRho*2))
      settings: SourceProductName=Simulink  SourceProductBaseCode=SL
  rd_data : Outport
  wires:
  rd_addr/1 -> Simple Dual Port RAM/4
  wr_en/1 -> Simple Dual Port RAM/3
  wr_addr/1 -> Simple Dual Port RAM/2
  wr_data/1 -> Simple Dual Port RAM/1
  Simple Dual Port RAM/1 -> rd_data/1

== system gm_parallel_lht/Parallel LHT/Parallel LHT Accumulator/Accumulator with Switches/Accumulator_instance62/Block RAM/Simple Dual Port RAM ==
  wr_data : Inport  OutDataTypeStr=fixdt(0, 11, 0)  PortDimensions=1  SampleTime=6.66666666666667e-09
  wr_addr : Inport  Port=2  OutDataTypeStr=fixdt(0, 11, 0)  PortDimensions=1  SampleTime=6.66666666666667e-09
  wr_en : Inport  Port=3  OutDataTypeStr=boolean  PortDimensions=1  SampleTime=6.66666666666667e-09
  rd_addr : Inport  Port=4  OutDataTypeStr=fixdt(0, 11, 0)  PortDimensions=1  SampleTime=6.66666666666667e-09
  Simple Dual Port RAM : hdlsllib/HDL RAMs/Simple Dual Port RAM  ram_size=ceil(log2(maxRho*2))
      settings: SourceProductName=Simulink  SourceProductBaseCode=SL
  rd_data : Outport
  wires:
  rd_addr/1 -> Simple Dual Port RAM/4
  wr_en/1 -> Simple Dual Port RAM/3
  wr_addr/1 -> Simple Dual Port RAM/2
  wr_data/1 -> Simple Dual Port RAM/1
  Simple Dual Port RAM/1 -> rd_data/1

== system gm_parallel_lht/Parallel LHT/Parallel LHT Accumulator/Accumulator with Switches/Accumulator_instance63/Block RAM/Simple Dual Port RAM ==
  wr_data : Inport  OutDataTypeStr=fixdt(0, 11, 0)  PortDimensions=1  SampleTime=6.66666666666667e-09
  wr_addr : Inport  Port=2  OutDataTypeStr=fixdt(0, 11, 0)  PortDimensions=1  SampleTime=6.66666666666667e-09
  wr_en : Inport  Port=3  OutDataTypeStr=boolean  PortDimensions=1  SampleTime=6.66666666666667e-09
  rd_addr : Inport  Port=4  OutDataTypeStr=fixdt(0, 11, 0)  PortDimensions=1  SampleTime=6.66666666666667e-09
  Simple Dual Port RAM : hdlsllib/HDL RAMs/Simple Dual Port RAM  ram_size=ceil(log2(maxRho*2))
      settings: SourceProductName=Simulink  SourceProductBaseCode=SL
  rd_data : Outport
  wires:
  rd_addr/1 -> Simple Dual Port RAM/4
  wr_en/1 -> Simple Dual Port RAM/3
  wr_addr/1 -> Simple Dual Port RAM/2
  wr_data/1 -> Simple Dual Port RAM/1
  Simple Dual Port RAM/1 -> rd_data/1

== system gm_parallel_lht/Parallel LHT/Parallel LHT Accumulator/Accumulator with Switches/Accumulator_instance64/Block RAM/Simple Dual Port RAM ==
  wr_data : Inport  OutDataTypeStr=fixdt(0, 11, 0)  PortDimensions=1  SampleTime=6.66666666666667e-09
  wr_addr : Inport  Port=2  OutDataTypeStr=fixdt(0, 11, 0)  PortDimensions=1  SampleTime=6.66666666666667e-09
  wr_en : Inport  Port=3  OutDataTypeStr=boolean  PortDimensions=1  SampleTime=6.66666666666667e-09
  rd_addr : Inport  Port=4  OutDataTypeStr=fixdt(0, 11, 0)  PortDimensions=1  SampleTime=6.66666666666667e-09
  Simple Dual Port RAM : hdlsllib/HDL RAMs/Simple Dual Port RAM  ram_size=ceil(log2(maxRho*2))
      settings: SourceProductName=Simulink  SourceProductBaseCode=SL
  rd_data : Outport
  wires:
  rd_addr/1 -> Simple Dual Port RAM/4
  wr_en/1 -> Simple Dual Port RAM/3
  wr_addr/1 -> Simple Dual Port RAM/2
  wr_data/1 -> Simple Dual Port RAM/1
  Simple Dual Port RAM/1 -> rd_data/1

== system gm_parallel_lht/Parallel LHT/Parallel LHT Accumulator/Accumulator with Switches/Accumulator_instance65/Block RAM/Simple Dual Port RAM ==
  wr_data : Inport  OutDataTypeStr=fixdt(0, 11, 0)  PortDimensions=1  SampleTime=6.66666666666667e-09
  wr_addr : Inport  Port=2  OutDataTypeStr=fixdt(0, 11, 0)  PortDimensions=1  SampleTime=6.66666666666667e-09
  wr_en : Inport  Port=3  OutDataTypeStr=boolean  PortDimensions=1  SampleTime=6.66666666666667e-09
  rd_addr : Inport  Port=4  OutDataTypeStr=fixdt(0, 11, 0)  PortDimensions=1  SampleTime=6.66666666666667e-09
  Simple Dual Port RAM : hdlsllib/HDL RAMs/Simple Dual Port RAM  ram_size=ceil(log2(maxRho*2))
      settings: SourceProductName=Simulink  SourceProductBaseCode=SL
  rd_data : Outport
  wires:
  rd_addr/1 -> Simple Dual Port RAM/4
  wr_en/1 -> Simple Dual Port RAM/3
  wr_addr/1 -> Simple Dual Port RAM/2
  wr_data/1 -> Simple Dual Port RAM/1
  Simple Dual Port RAM/1 -> rd_data/1

== system gm_parallel_lht/Parallel LHT/Parallel LHT Accumulator/Accumulator with Switches/Accumulator_instance66/Block RAM/Simple Dual Port RAM ==
  wr_data : Inport  OutDataTypeStr=fixdt(0, 11, 0)  PortDimensions=1  SampleTime=6.66666666666667e-09
  wr_addr : Inport  Port=2  OutDataTypeStr=fixdt(0, 11, 0)  PortDimensions=1  SampleTime=6.66666666666667e-09
  wr_en : Inport  Port=3  OutDataTypeStr=boolean  PortDimensions=1  SampleTime=6.66666666666667e-09
  rd_addr : Inport  Port=4  OutDataTypeStr=fixdt(0, 11, 0)  PortDimensions=1  SampleTime=6.66666666666667e-09
  Simple Dual Port RAM : hdlsllib/HDL RAMs/Simple Dual Port RAM  ram_size=ceil(log2(maxRho*2))
      settings: SourceProductName=Simulink  SourceProductBaseCode=SL
  rd_data : Outport
  wires:
  rd_addr/1 -> Simple Dual Port RAM/4
  wr_en/1 -> Simple Dual Port RAM/3
  wr_addr/1 -> Simple Dual Port RAM/2
  wr_data/1 -> Simple Dual Port RAM/1
  Simple Dual Port RAM/1 -> rd_data/1

== system gm_parallel_lht/Parallel LHT/Parallel LHT Accumulator/Accumulator with Switches/Accumulator_instance67/Block RAM/Simple Dual Port RAM ==
  wr_data : Inport  OutDataTypeStr=fixdt(0, 11, 0)  PortDimensions=1  SampleTime=6.66666666666667e-09
  wr_addr : Inport  Port=2  OutDataTypeStr=fixdt(0, 11, 0)  PortDimensions=1  SampleTime=6.66666666666667e-09
  wr_en : Inport  Port=3  OutDataTypeStr=boolean  PortDimensions=1  SampleTime=6.66666666666667e-09
  rd_addr : Inport  Port=4  OutDataTypeStr=fixdt(0, 11, 0)  PortDimensions=1  SampleTime=6.66666666666667e-09
  Simple Dual Port RAM : hdlsllib/HDL RAMs/Simple Dual Port RAM  ram_size=ceil(log2(maxRho*2))
      settings: SourceProductName=Simulink  SourceProductBaseCode=SL
  rd_data : Outport
  wires:
  rd_addr/1 -> Simple Dual Port RAM/4
  wr_en/1 -> Simple Dual Port RAM/3
  wr_addr/1 -> Simple Dual Port RAM/2
  wr_data/1 -> Simple Dual Port RAM/1
  Simple Dual Port RAM/1 -> rd_data/1

== system gm_parallel_lht/Parallel LHT/Parallel LHT Accumulator/Accumulator with Switches/Accumulator_instance68/Block RAM/Simple Dual Port RAM ==
  wr_data : Inport  OutDataTypeStr=fixdt(0, 11, 0)  PortDimensions=1  SampleTime=6.66666666666667e-09
  wr_addr : Inport  Port=2  OutDataTypeStr=fixdt(0, 11, 0)  PortDimensions=1  SampleTime=6.66666666666667e-09
  wr_en : Inport  Port=3  OutDataTypeStr=boolean  PortDimensions=1  SampleTime=6.66666666666667e-09
  rd_addr : Inport  Port=4  OutDataTypeStr=fixdt(0, 11, 0)  PortDimensions=1  SampleTime=6.66666666666667e-09
  Simple Dual Port RAM : hdlsllib/HDL RAMs/Simple Dual Port RAM  ram_size=ceil(log2(maxRho*2))
      settings: SourceProductName=Simulink  SourceProductBaseCode=SL
  rd_data : Outport
  wires:
  rd_addr/1 -> Simple Dual Port RAM/4
  wr_en/1 -> Simple Dual Port RAM/3
  wr_addr/1 -> Simple Dual Port RAM/2
  wr_data/1 -> Simple Dual Port RAM/1
  Simple Dual Port RAM/1 -> rd_data/1

== system gm_parallel_lht/Parallel LHT/Parallel LHT Accumulator/Accumulator with Switches/Accumulator_instance69/Block RAM/Simple Dual Port RAM ==
  wr_data : Inport  OutDataTypeStr=fixdt(0, 11, 0)  PortDimensions=1  SampleTime=6.66666666666667e-09
  wr_addr : Inport  Port=2  OutDataTypeStr=fixdt(0, 11, 0)  PortDimensions=1  SampleTime=6.66666666666667e-09
  wr_en : Inport  Port=3  OutDataTypeStr=boolean  PortDimensions=1  SampleTime=6.66666666666667e-09
  rd_addr : Inport  Port=4  OutDataTypeStr=fixdt(0, 11, 0)  PortDimensions=1  SampleTime=6.66666666666667e-09
  Simple Dual Port RAM : hdlsllib/HDL RAMs/Simple Dual Port RAM  ram_size=ceil(log2(maxRho*2))
      settings: SourceProductName=Simulink  SourceProductBaseCode=SL
  rd_data : Outport
  wires:
  rd_addr/1 -> Simple Dual Port RAM/4
  wr_en/1 -> Simple Dual Port RAM/3
  wr_addr/1 -> Simple Dual Port RAM/2
  wr_data/1 -> Simple Dual Port RAM/1
  Simple Dual Port RAM/1 -> rd_data/1

== system gm_parallel_lht/Parallel LHT/Parallel LHT Accumulator/Accumulator with Switches/Accumulator_instance7/Block RAM/Simple Dual Port RAM ==
  wr_data : Inport  OutDataTypeStr=fixdt(0, 11, 0)  PortDimensions=1  SampleTime=6.66666666666667e-09
  wr_addr : Inport  Port=2  OutDataTypeStr=fixdt(0, 11, 0)  PortDimensions=1  SampleTime=6.66666666666667e-09
  wr_en : Inport  Port=3  OutDataTypeStr=boolean  PortDimensions=1  SampleTime=6.66666666666667e-09
  rd_addr : Inport  Port=4  OutDataTypeStr=fixdt(0, 11, 0)  PortDimensions=1  SampleTime=6.66666666666667e-09
  Simple Dual Port RAM : hdlsllib/HDL RAMs/Simple Dual Port RAM  ram_size=ceil(log2(maxRho*2))
      settings: SourceProductName=Simulink  SourceProductBaseCode=SL
  rd_data : Outport
  wires:
  rd_addr/1 -> Simple Dual Port RAM/4
  wr_en/1 -> Simple Dual Port RAM/3
  wr_addr/1 -> Simple Dual Port RAM/2
  wr_data/1 -> Simple Dual Port RAM/1
  Simple Dual Port RAM/1 -> rd_data/1

== system gm_parallel_lht/Parallel LHT/Parallel LHT Accumulator/Accumulator with Switches/Accumulator_instance70/Block RAM/Simple Dual Port RAM ==
  wr_data : Inport  OutDataTypeStr=fixdt(0, 11, 0)  PortDimensions=1  SampleTime=6.66666666666667e-09
  wr_addr : Inport  Port=2  OutDataTypeStr=fixdt(0, 11, 0)  PortDimensions=1  SampleTime=6.66666666666667e-09
  wr_en : Inport  Port=3  OutDataTypeStr=boolean  PortDimensions=1  SampleTime=6.66666666666667e-09
  rd_addr : Inport  Port=4  OutDataTypeStr=fixdt(0, 11, 0)  PortDimensions=1  SampleTime=6.66666666666667e-09
  Simple Dual Port RAM : hdlsllib/HDL RAMs/Simple Dual Port RAM  ram_size=ceil(log2(maxRho*2))
      settings: SourceProductName=Simulink  SourceProductBaseCode=SL
  rd_data : Outport
  wires:
  rd_addr/1 -> Simple Dual Port RAM/4
  wr_en/1 -> Simple Dual Port RAM/3
  wr_addr/1 -> Simple Dual Port RAM/2
  wr_data/1 -> Simple Dual Port RAM/1
  Simple Dual Port RAM/1 -> rd_data/1

== system gm_parallel_lht/Parallel LHT/Parallel LHT Accumulator/Accumulator with Switches/Accumulator_instance71/Block RAM/Simple Dual Port RAM ==
  wr_data : Inport  OutDataTypeStr=fixdt(0, 11, 0)  PortDimensions=1  SampleTime=6.66666666666667e-09
  wr_addr : Inport  Port=2  OutDataTypeStr=fixdt(0, 11, 0)  PortDimensions=1  SampleTime=6.66666666666667e-09
  wr_en : Inport  Port=3  OutDataTypeStr=boolean  PortDimensions=1  SampleTime=6.66666666666667e-09
  rd_addr : Inport  Port=4  OutDataTypeStr=fixdt(0, 11, 0)  PortDimensions=1  SampleTime=6.66666666666667e-09
  Simple Dual Port RAM : hdlsllib/HDL RAMs/Simple Dual Port RAM  ram_size=ceil(log2(maxRho*2))
      settings: SourceProductName=Simulink  SourceProductBaseCode=SL
  rd_data : Outport
  wires:
  rd_addr/1 -> Simple Dual Port RAM/4
  wr_en/1 -> Simple Dual Port RAM/3
  wr_addr/1 -> Simple Dual Port RAM/2
  wr_data/1 -> Simple Dual Port RAM/1
  Simple Dual Port RAM/1 -> rd_data/1

== system gm_parallel_lht/Parallel LHT/Parallel LHT Accumulator/Accumulator with Switches/Accumulator_instance72/Block RAM/Simple Dual Port RAM ==
  wr_data : Inport  OutDataTypeStr=fixdt(0, 11, 0)  PortDimensions=1  SampleTime=6.66666666666667e-09
  wr_addr : Inport  Port=2  OutDataTypeStr=fixdt(0, 11, 0)  PortDimensions=1  SampleTime=6.66666666666667e-09
  wr_en : Inport  Port=3  OutDataTypeStr=boolean  PortDimensions=1  SampleTime=6.66666666666667e-09
  rd_addr : Inport  Port=4  OutDataTypeStr=fixdt(0, 11, 0)  PortDimensions=1  SampleTime=6.66666666666667e-09
  Simple Dual Port RAM : hdlsllib/HDL RAMs/Simple Dual Port RAM  ram_size=ceil(log2(maxRho*2))
      settings: SourceProductName=Simulink  SourceProductBaseCode=SL
  rd_data : Outport
  wires:
  rd_addr/1 -> Simple Dual Port RAM/4
  wr_en/1 -> Simple Dual Port RAM/3
  wr_addr/1 -> Simple Dual Port RAM/2
  wr_data/1 -> Simple Dual Port RAM/1
  Simple Dual Port RAM/1 -> rd_data/1

== system gm_parallel_lht/Parallel LHT/Parallel LHT Accumulator/Accumulator with Switches/Accumulator_instance73/Block RAM/Simple Dual Port RAM ==
  wr_data : Inport  OutDataTypeStr=fixdt(0, 11, 0)  PortDimensions=1  SampleTime=6.66666666666667e-09
  wr_addr : Inport  Port=2  OutDataTypeStr=fixdt(0, 11, 0)  PortDimensions=1  SampleTime=6.66666666666667e-09
  wr_en : Inport  Port=3  OutDataTypeStr=boolean  PortDimensions=1  SampleTime=6.66666666666667e-09
  rd_addr : Inport  Port=4  OutDataTypeStr=fixdt(0, 11, 0)  PortDimensions=1  SampleTime=6.66666666666667e-09
  Simple Dual Port RAM : hdlsllib/HDL RAMs/Simple Dual Port RAM  ram_size=ceil(log2(maxRho*2))
      settings: SourceProductName=Simulink  SourceProductBaseCode=SL
  rd_data : Outport
  wires:
  rd_addr/1 -> Simple Dual Port RAM/4
  wr_en/1 -> Simple Dual Port RAM/3
  wr_addr/1 -> Simple Dual Port RAM/2
  wr_data/1 -> Simple Dual Port RAM/1
  Simple Dual Port RAM/1 -> rd_data/1

== system gm_parallel_lht/Parallel LHT/Parallel LHT Accumulator/Accumulator with Switches/Accumulator_instance74/Block RAM/Simple Dual Port RAM ==
  wr_data : Inport  OutDataTypeStr=fixdt(0, 11, 0)  PortDimensions=1  SampleTime=6.66666666666667e-09
  wr_addr : Inport  Port=2  OutDataTypeStr=fixdt(0, 11, 0)  PortDimensions=1  SampleTime=6.66666666666667e-09
  wr_en : Inport  Port=3  OutDataTypeStr=boolean  PortDimensions=1  SampleTime=6.66666666666667e-09
  rd_addr : Inport  Port=4  OutDataTypeStr=fixdt(0, 11, 0)  PortDimensions=1  SampleTime=6.66666666666667e-09
  Simple Dual Port RAM : hdlsllib/HDL RAMs/Simple Dual Port RAM  ram_size=ceil(log2(maxRho*2))
      settings: SourceProductName=Simulink  SourceProductBaseCode=SL
  rd_data : Outport
  wires:
  rd_addr/1 -> Simple Dual Port RAM/4
  wr_en/1 -> Simple Dual Port RAM/3
  wr_addr/1 -> Simple Dual Port RAM/2
  wr_data/1 -> Simple Dual Port RAM/1
  Simple Dual Port RAM/1 -> rd_data/1

== system gm_parallel_lht/Parallel LHT/Parallel LHT Accumulator/Accumulator with Switches/Accumulator_instance75/Block RAM/Simple Dual Port RAM ==
  wr_data : Inport  OutDataTypeStr=fixdt(0, 11, 0)  PortDimensions=1  SampleTime=6.66666666666667e-09
  wr_addr : Inport  Port=2  OutDataTypeStr=fixdt(0, 11, 0)  PortDimensions=1  SampleTime=6.66666666666667e-09
  wr_en : Inport  Port=3  OutDataTypeStr=boolean  PortDimensions=1  SampleTime=6.66666666666667e-09
  rd_addr : Inport  Port=4  OutDataTypeStr=fixdt(0, 11, 0)  PortDimensions=1  SampleTime=6.66666666666667e-09
  Simple Dual Port RAM : hdlsllib/HDL RAMs/Simple Dual Port RAM  ram_size=ceil(log2(maxRho*2))
      settings: SourceProductName=Simulink  SourceProductBaseCode=SL
  rd_data : Outport
  wires:
  rd_addr/1 -> Simple Dual Port RAM/4
  wr_en/1 -> Simple Dual Port RAM/3
  wr_addr/1 -> Simple Dual Port RAM/2
  wr_data/1 -> Simple Dual Port RAM/1
  Simple Dual Port RAM/1 -> rd_data/1

== system gm_parallel_lht/Parallel LHT/Parallel LHT Accumulator/Accumulator with Switches/Accumulator_instance76/Block RAM/Simple Dual Port RAM ==
  wr_data : Inport  OutDataTypeStr=fixdt(0, 11, 0)  PortDimensions=1  SampleTime=6.66666666666667e-09
  wr_addr : Inport  Port=2  OutDataTypeStr=fixdt(0, 11, 0)  PortDimensions=1  SampleTime=6.66666666666667e-09
  wr_en : Inport  Port=3  OutDataTypeStr=boolean  PortDimensions=1  SampleTime=6.66666666666667e-09
  rd_addr : Inport  Port=4  OutDataTypeStr=fixdt(0, 11, 0)  PortDimensions=1  SampleTime=6.66666666666667e-09
  Simple Dual Port RAM : hdlsllib/HDL RAMs/Simple Dual Port RAM  ram_size=ceil(log2(maxRho*2))
      settings: SourceProductName=Simulink  SourceProductBaseCode=SL
  rd_data : Outport
  wires:
  rd_addr/1 -> Simple Dual Port RAM/4
  wr_en/1 -> Simple Dual Port RAM/3
  wr_addr/1 -> Simple Dual Port RAM/2
  wr_data/1 -> Simple Dual Port RAM/1
  Simple Dual Port RAM/1 -> rd_data/1

== system gm_parallel_lht/Parallel LHT/Parallel LHT Accumulator/Accumulator with Switches/Accumulator_instance77/Block RAM/Simple Dual Port RAM ==
  wr_data : Inport  OutDataTypeStr=fixdt(0, 11, 0)  PortDimensions=1  SampleTime=6.66666666666667e-09
  wr_addr : Inport  Port=2  OutDataTypeStr=fixdt(0, 11, 0)  PortDimensions=1  SampleTime=6.66666666666667e-09
  wr_en : Inport  Port=3  OutDataTypeStr=boolean  PortDimensions=1  SampleTime=6.66666666666667e-09
  rd_addr : Inport  Port=4  OutDataTypeStr=fixdt(0, 11, 0)  PortDimensions=1  SampleTime=6.66666666666667e-09
  Simple Dual Port RAM : hdlsllib/HDL RAMs/Simple Dual Port RAM  ram_size=ceil(log2(maxRho*2))
      settings: SourceProductName=Simulink  SourceProductBaseCode=SL
  rd_data : Outport
  wires:
  rd_addr/1 -> Simple Dual Port RAM/4
  wr_en/1 -> Simple Dual Port RAM/3
  wr_addr/1 -> Simple Dual Port RAM/2
  wr_data/1 -> Simple Dual Port RAM/1
  Simple Dual Port RAM/1 -> rd_data/1

== system gm_parallel_lht/Parallel LHT/Parallel LHT Accumulator/Accumulator with Switches/Accumulator_instance78/Block RAM/Simple Dual Port RAM ==
  wr_data : Inport  OutDataTypeStr=fixdt(0, 11, 0)  PortDimensions=1  SampleTime=6.66666666666667e-09
  wr_addr : Inport  Port=2  OutDataTypeStr=fixdt(0, 11, 0)  PortDimensions=1  SampleTime=6.66666666666667e-09
  wr_en : Inport  Port=3  OutDataTypeStr=boolean  PortDimensions=1  SampleTime=6.66666666666667e-09
  rd_addr : Inport  Port=4  OutDataTypeStr=fixdt(0, 11, 0)  PortDimensions=1  SampleTime=6.66666666666667e-09
  Simple Dual Port RAM : hdlsllib/HDL RAMs/Simple Dual Port RAM  ram_size=ceil(log2(maxRho*2))
      settings: SourceProductName=Simulink  SourceProductBaseCode=SL
  rd_data : Outport
  wires:
  rd_addr/1 -> Simple Dual Port RAM/4
  wr_en/1 -> Simple Dual Port RAM/3
  wr_addr/1 -> Simple Dual Port RAM/2
  wr_data/1 -> Simple Dual Port RAM/1
  Simple Dual Port RAM/1 -> rd_data/1

== system gm_parallel_lht/Parallel LHT/Parallel LHT Accumulator/Accumulator with Switches/Accumulator_instance79/Block RAM/Simple Dual Port RAM ==
  wr_data : Inport  OutDataTypeStr=fixdt(0, 11, 0)  PortDimensions=1  SampleTime=6.66666666666667e-09
  wr_addr : Inport  Port=2  OutDataTypeStr=fixdt(0, 11, 0)  PortDimensions=1  SampleTime=6.66666666666667e-09
  wr_en : Inport  Port=3  OutDataTypeStr=boolean  PortDimensions=1  SampleTime=6.66666666666667e-09
  rd_addr : Inport  Port=4  OutDataTypeStr=fixdt(0, 11, 0)  PortDimensions=1  SampleTime=6.66666666666667e-09
  Simple Dual Port RAM : hdlsllib/HDL RAMs/Simple Dual Port RAM  ram_size=ceil(log2(maxRho*2))
      settings: SourceProductName=Simulink  SourceProductBaseCode=SL
  rd_data : Outport
  wires:
  rd_addr/1 -> Simple Dual Port RAM/4
  wr_en/1 -> Simple Dual Port RAM/3
  wr_addr/1 -> Simple Dual Port RAM/2
  wr_data/1 -> Simple Dual Port RAM/1
  Simple Dual Port RAM/1 -> rd_data/1

== system gm_parallel_lht/Parallel LHT/Parallel LHT Accumulator/Accumulator with Switches/Accumulator_instance8/Block RAM/Simple Dual Port RAM ==
  wr_data : Inport  OutDataTypeStr=fixdt(0, 11, 0)  PortDimensions=1  SampleTime=6.66666666666667e-09
  wr_addr : Inport  Port=2  OutDataTypeStr=fixdt(0, 11, 0)  PortDimensions=1  SampleTime=6.66666666666667e-09
  wr_en : Inport  Port=3  OutDataTypeStr=boolean  PortDimensions=1  SampleTime=6.66666666666667e-09
  rd_addr : Inport  Port=4  OutDataTypeStr=fixdt(0, 11, 0)  PortDimensions=1  SampleTime=6.66666666666667e-09
  Simple Dual Port RAM : hdlsllib/HDL RAMs/Simple Dual Port RAM  ram_size=ceil(log2(maxRho*2))
      settings: SourceProductName=Simulink  SourceProductBaseCode=SL
  rd_data : Outport
  wires:
  rd_addr/1 -> Simple Dual Port RAM/4
  wr_en/1 -> Simple Dual Port RAM/3
  wr_addr/1 -> Simple Dual Port RAM/2
  wr_data/1 -> Simple Dual Port RAM/1
  Simple Dual Port RAM/1 -> rd_data/1

== system gm_parallel_lht/Parallel LHT/Parallel LHT Accumulator/Accumulator with Switches/Accumulator_instance80/Block RAM/Simple Dual Port RAM ==
  wr_data : Inport  OutDataTypeStr=fixdt(0, 11, 0)  PortDimensions=1  SampleTime=6.66666666666667e-09
  wr_addr : Inport  Port=2  OutDataTypeStr=fixdt(0, 11, 0)  PortDimensions=1  SampleTime=6.66666666666667e-09
  wr_en : Inport  Port=3  OutDataTypeStr=boolean  PortDimensions=1  SampleTime=6.66666666666667e-09
  rd_addr : Inport  Port=4  OutDataTypeStr=fixdt(0, 11, 0)  PortDimensions=1  SampleTime=6.66666666666667e-09
  Simple Dual Port RAM : hdlsllib/HDL RAMs/Simple Dual Port RAM  ram_size=ceil(log2(maxRho*2))
      settings: SourceProductName=Simulink  SourceProductBaseCode=SL
  rd_data : Outport
  wires:
  rd_addr/1 -> Simple Dual Port RAM/4
  wr_en/1 -> Simple Dual Port RAM/3
  wr_addr/1 -> Simple Dual Port RAM/2
  wr_data/1 -> Simple Dual Port RAM/1
  Simple Dual Port RAM/1 -> rd_data/1

== system gm_parallel_lht/Parallel LHT/Parallel LHT Accumulator/Accumulator with Switches/Accumulator_instance81/Block RAM/Simple Dual Port RAM ==
  wr_data : Inport  OutDataTypeStr=fixdt(0, 11, 0)  PortDimensions=1  SampleTime=6.66666666666667e-09
  wr_addr : Inport  Port=2  OutDataTypeStr=fixdt(0, 11, 0)  PortDimensions=1  SampleTime=6.66666666666667e-09
  wr_en : Inport  Port=3  OutDataTypeStr=boolean  PortDimensions=1  SampleTime=6.66666666666667e-09
  rd_addr : Inport  Port=4  OutDataTypeStr=fixdt(0, 11, 0)  PortDimensions=1  SampleTime=6.66666666666667e-09
  Simple Dual Port RAM : hdlsllib/HDL RAMs/Simple Dual Port RAM  ram_size=ceil(log2(maxRho*2))
      settings: SourceProductName=Simulink  SourceProductBaseCode=SL
  rd_data : Outport
  wires:
  rd_addr/1 -> Simple Dual Port RAM/4
  wr_en/1 -> Simple Dual Port RAM/3
  wr_addr/1 -> Simple Dual Port RAM/2
  wr_data/1 -> Simple Dual Port RAM/1
  Simple Dual Port RAM/1 -> rd_data/1
